simulink model "Case_SPM"  (R2026a)
settings: Solver=ode15s  StopTime=108000  RelTol=1e-6  AbsTol=1e-7
InitFcn:
  | parameters_reference
libraries: simulink x3, fl_lib x3, nesl_utility x3, batt_lib x1
settings Model: Creator=gurha  LastModifiedBy=gurha

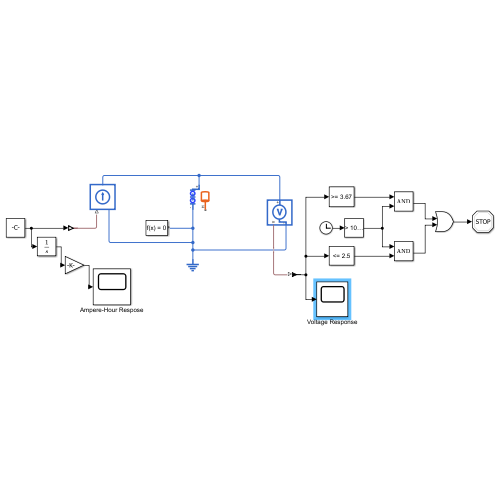
[thumbnail: Simulink's stored preview of the top-level diagram]
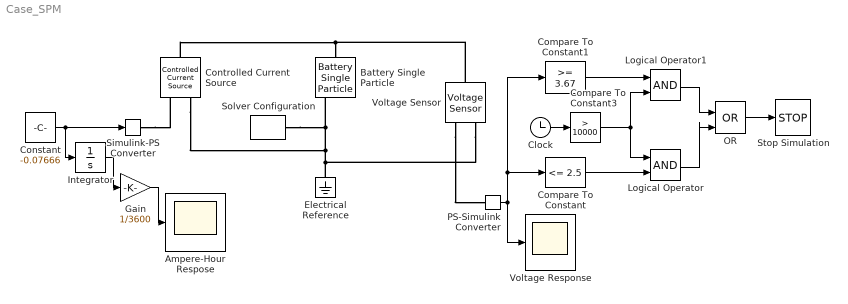
== system Case_SPM ==
  Ampere-Hour Respose : Scope
      settings: ActiveDisplayYMinimum=-2.4807214951874759  ActiveDisplayYMaximum=0.37180241892208388
  Battery Single Particle : batt_lib/Cells/Electrochemical/Battery Single Particle  ExtrapolationMethod=simscape.enum.extrapolation.nearest  ThicknessAnode=3.4e-5 m  ElectrolyteLayerCountAnode=10  ThicknessSeparator=3E-5 m  ElectrolyteLayerCountSeparator=5  ThicknessCathode=7E-5 m  ElectrolyteLayerCountCathode=10  ElectrodePlateArea=0.1755 m^2  ParticleRadiusAnode=3.5E-6 m  ShellCountAnode=10  ParticleRadiusCathode=3.65E-8 m  ShellCountCathode=10  ActiveMaterialVolumeFractionAnode=0.55  ActiveMaterialVolumeFractionCathode=0.43  StoichiometryBreakpointsSpecification=simscape.battery.enum.cells.electrochemical.StoichiometryBreakpointsSpecification.normalized  NormalizedStoichiometryBreakpoints=x_vec  OpenCircuitPotentialAnode=U_anode V  OpenCircuitPotentialCathode=U_cathode V  AbsoluteStoichiometryBreakpointsAnode=linspace(0.025, 0.975, 39)  OpenCircuitPotentialAbsoluteAnode=[.484; .335; .253; .209; .2; .181; .165; .151; .139; .131; .128; .125; .124; .124; .123; .122; .119; .117; .111; .108; .101; .098; .095; .093; .092; .088; .088; .088; .088; .087; .087; .087; .085; .082; .079; .071; .064; .049; .026] V  AbsoluteStoichiometryBreakpointsCathode=linspace(0.025, 0.975, 39)  OpenCircuitPotentialAbsoluteCathode=[3.81; 3.608; 3.512; 3.478; 3.459; 3.453; 3.45257; 3.45214; 3.45171; 3.45128; 3.45085; 3.45042; 3.44999; 3.44956; 3.44913; 3.4487; 3.44827; 3.44784; 3.44741; 3.44698; 3.44655; 3.44612; 3.44569; 3.44526; 3.44483; 3.4444; 3.44397; 3.44354; 3.44311; 3.44268; 3.44225; 3.44182; 3.44139; 3.44096; 3.44053; 3.44; 3.412; 3.304; 2.968] V  MaximumConcentrationAnode=31370 mol/m^3  MaximumStoichiometryAnode=0.8320  MinimumStoichiometryAnode=0.0072  MaximumConcentrationCathode=22806 mol/m^3  MaximumStoichiometryCathode=0.9822  MinimumStoichiometryCathode=0.06  ActiveMaterialDiffusionCoefficientAnode=1.3E-16 m^2/s  ActiveMaterialDiffusionCoefficientCathode=2.7E-14 m^2/s  ConductivityAnode=100 S/m  ConductivityCathode=0.5 S/m  CurrentCollectorResistance=38.5e-3 Ohm  ElectrolyteVolumeFractionAnode=0.33  ElectrolyteVolumeFractionSeparator=0.54  ElectrolyteVolumeFractionCathode=0.332  ElectrolyteConductivity=0.2 S/m  BruggemanExponentAnode=1.5  BruggemanExponentSeparator=1.5  BruggemanExponentCathode=1.5  TransferenceNumber=0.363  ElectrolyteDiffusionCoefficient=2E-10 m^2/s  ChargeTransferRateAnode=3.9E-10 m^(5/2)/(mol^(1/2)*s)  ChargeTransferRateCathode=1.1E-11 m^(5/2)/(mol^(1/2)*s)  BatteryThermalMass=77 J/K  ArrheniusReferenceTemperature=298.15 K  ActiveMaterialDiffusionActivationEnergyAnode=39000 J/mol  ActiveMaterialDiffusionActivationEnergyCathode=35000 J/mol  ElectrolyteDiffusionActivationEnergy=26600 J/mol  ConductivityActivationEnergyAnode=3000 J/mol  ConductivityActivationEnergyCathode=3000 J/mol  ElectrolyteConductivityActivationEnergy=11000 J/mol  ChargeTransferActivationEnergyAnode=13000 J/mol  ChargeTransferActivationEnergyCathode=20000 J/mol  InnerSEIMethod=simscape.battery.enum.cells.electrochemical.InnerSEIMethod.diffusionLimitedSEIGrowth  MolarVolumeInnerSEI=5E-3 m^3/mol  DiffusionCoefficientInnerSEI=1E-20 m^2/s  StoichiometricCoefficientInnerSEI=2  DiffusionActivationEnergyInnerSEI=39000 J/mol  ConductivityInnerSEI=5.0E-6 S/m  ConductivityActivationEnergyInnerSEI=39000 J/mol  PlatingMethod=simscape.battery.enum.cells.electrochemical.PlatingMethod.none  ExchangeCurrentDensityPlating=3E-4 A/m^2  ActivationEnergyPlating=3000 J/mol  ReversibilityFactorPlating=0.5  batteryCurrent_specify=off  batteryCurrent_priority=None  batteryCurrent=0 A  batteryCurrent_nominal_specify=off  batteryCurrent_nominal_value=1  batteryCurrent_nominal_unit=A  batteryVoltage_specify=off  batteryVoltage_priority=None  batteryVoltage=0 V  batteryVoltage_nominal_specify=off  batteryVoltage_nominal_value=1  batteryVoltage_nominal_unit=V  averageElectrolyteConcentration_specify=off  averageElectrolyteConcentration_priority=High  averageElectrolyteConcentration=1200 mol/m^3  averageElectrolyteConcentration_nominal_specify=off  averageElectrolyteConcentration_nominal_value=1  averageElectrolyteConcentration_nominal_unit=mol/m^3  stateOfCharge_specify=on  stateOfCharge_priority=High  stateOfCharge=1  stateOfCharge_nominal_specify=off  stateOfCharge_nominal_value=1  stateOfCharge_nominal_unit=1  batteryTemperature_specify=off  batteryTemperature_priority=High  batteryTemperature=298.15 K  batteryTemperature_nominal_specify=off  batteryTemperature_nominal_value=1  batteryTemperature_nominal_unit=K  thicknessSEI_specify=off  thicknessSEI_priority=High  thicknessSEI=1E-7 m  thicknessSEI_nominal_specify=off  thicknessSEI_nominal_value=1  thicknessSEI_nominal_unit=m  reversiblePlatedMaterial_specify=off  reversiblePlatedMaterial_priority=High  reversiblePlatedMaterial=0 mol  reversiblePlatedMaterial_nominal_specify=off  reversiblePlatedMaterial_nominal_value=1  reversiblePlatedMaterial_nominal_unit=mol  irreversiblePlatedMaterial_specify=off  irreversiblePlatedMaterial_priority=High  irreversiblePlatedMaterial=0 mol  irreversiblePlatedMaterial_nominal_specify=off  irreversiblePlatedMaterial_nominal_value=1  irreversiblePlatedMaterial_nominal_unit=mol  power_dissipated_specify=off  power_dissipated_priority=None  power_dissipated=0 W  power_dissipated_nominal_specify=off  power_dissipated_nominal_value=1  power_dissipated_nominal_unit=W  heatGenerationRate_specify=off  heatGenerationRate_priority=None  heatGenerationRate=0 W  heatGenerationRate_nominal_specify=off  heatGenerationRate_nominal_value=1  heatGenerationRate_nominal_unit=W
  Clock : Clock
      settings: Decimation=1000
  Compare To Constant : simulink/Logic and Bit Operations/Compare To Constant  relop=<=  const=2.5  OutDataTypeStr=boolean
  Compare To Constant1 : simulink/Logic and Bit Operations/Compare To Constant  relop=>=  const=3.67  OutDataTypeStr=boolean
  Compare To Constant3 : simulink/Logic and Bit Operations/Compare To Constant  relop=>  const=10000  OutDataTypeStr=boolean
  Constant : Constant  Value=-0.07666
  Controlled Current Source : fl_lib/Electrical/Electrical Sources/Controlled Current Source
  Electrical Reference : fl_lib/Electrical/Electrical Elements/Electrical Reference
  Gain : Gain  Gain=1/3600
  Integrator : Integrator
  Logical Operator : Logic  AllPortsSameDT=off  OutDataTypeStr=boolean
  Logical Operator1 : Logic  AllPortsSameDT=off  OutDataTypeStr=boolean
  OR : Logic  Operator=OR  IconShape=distinctive  AllPortsSameDT=off  OutDataTypeStr=boolean
  PS-Simulink Converter : nesl_utility/PS-Simulink Converter  PhysicalDomain=network_engine_domain  SubClassName=ps_output  LeftPortType=input  RightPortType=output  PseudoPeriodic=off  Frequencies=[]  VectorFormat=inherit  Unit=inherit  AffineConversion=off
  Simulink-PS Converter : nesl_utility/Simulink-PS Converter  PhysicalDomain=network_engine_domain  SubClassName=ps_input  LeftPortType=input  RightPortType=output  PseudoPeriodic=off  Frequencies=[]  NoiseDistribution=none  NoiseParameters=[]  Unit=1  AffineConversion=off  FilteringAndDerivatives=provide  SimscapeFilterOrder=1  InputFilterTimeConstant=0.001  UdotUserProvided=0
  Solver Configuration : nesl_utility/Solver Configuration  PhysicalDomain=network_engine_domain  SubClassName=solver  LeftPortType=input  RightPortType=generic  Tones=[]  Harmonics=[]  SimulateNoise=off  Profile=off  UseLocalSampling=off  EnableSwitchedLinearOptims=on  FrequencyDomain=off  UseCCode=off  RelTol=0.001  AbsTol=0.001  MinStep=1e-09  ToWorkspace=off  RevertToSquareIcSolve=off  NumHomotopyIterations=100  PhasorMode=off  PhasorModeNumHarmonics=1  ConsistencySolver=NEWTON_XTOL_AFTER_FTOL  CanonicalOrdering=CANONICAL  OptimizeIntermediates=OPTIMIZED  IndexReductionMethod=DerivativeReplacement  DoDC=off  ResidualTolerance=1e-09  ConsistencyTolSource=GLOBAL  ConsistencyAbsTol=0.001  ConsistencyRelTol=0.001  ConsistencyTolFactor=1e-6  UseLocalSolver=off  LocalSolverChoice=NE_BACKWARD_EULER_ADVANCER  ResolveIndetEquations=on  FunctionEvalNumThread=1  LocalSolverSampleTime=0.001  DoFixedCost=off  MaxNonlinIter=3  MaxModeIter=2  ComputeImpulses=off  ImpulseIterations=2  LinearAlgebra=auto  LinearAlgebraNumThread=0  EquationFormulation=NE_TIME_EF  DelaysMemoryBudget=1024  AutomaticFiltering=on  FilteringTimeConstant=0.001  PartitionStorageMethod=AS_NEEDED  PartitionMemoryBudget=1024  PartitionMethod=ROBUST  MultibodyUseLocalSolver=off  MultibodyLocalSolverChoice=ODE1  MultibodyLocalSolverSampleTime=0.001
  Stop Simulation : Stop
  Voltage Response : Scope
      settings: ActiveDisplayYMinimum=2.2914582672840815  ActiveDisplayYMaximum=4.0868380069990176
  Voltage Sensor : fl_lib/Electrical/Electrical Sensors/Voltage Sensor
  wires:
  Constant/1 -> Simulink-PS Converter/1, Integrator/1
  PS-Simulink Converter/1 -> Compare To Constant1/1, Compare To Constant/1, Voltage Response/1
  Integrator/1 -> Gain/1
  Gain/1 -> Ampere-Hour Respose/1
  Compare To Constant/1 -> Logical Operator/2
  Clock/1 -> Compare To Constant3/1
  Logical Operator/1 -> OR/2
  Compare To Constant1/1 -> Logical Operator1/1
  Compare To Constant3/1 -> Logical Operator/1, Logical Operator1/2
  Logical Operator1/1 -> OR/1
  OR/1 -> Stop Simulation/1
  connections:
  Electrical Reference/LConn1 -- Voltage Sensor/RConn2 -- Battery Single Particle/RConn1 -- Solver Configuration/RConn1 -- Controlled Current Source/RConn2
  Controlled Current Source/LConn1 -- Voltage Sensor/LConn1 -- Battery Single Particle/LConn1
  Simulink-PS Converter/RConn1 -- Controlled Current Source/RConn1
  Voltage Sensor/RConn1 -- PS-Simulink Converter/LConn1
